simulink library "MET_lib"  (R2016b)
settings: Solver=VariableStepAuto  StartTime=0.0  StopTime=10.0  RelTol=1e-3
undefined symbols (not defined in the file or in its folder): sim_params
settings Model: Creator=taylorreynolds  LastModifiedBy=taylorreynolds

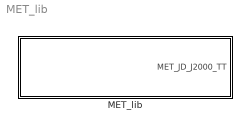
== system MET_lib ==
  MET_lib : Subsystem

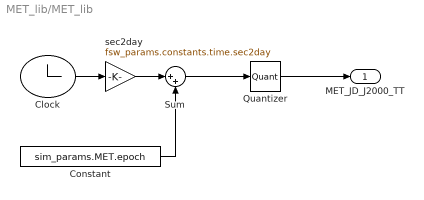
== system MET_lib/MET_lib ==
  Clock : Clock
  Constant : Constant  Value=sim_params.MET.epoch
  Quantizer : Quantizer  QuantizationInterval=sim_params.MET.res
  Sum : Sum  Inputs=|++
  sec2day : Gain  Gain=fsw_params.constants.time.sec2day
  MET_JD_J2000_TT : Outport
  wires:
  Clock/1 -> sec2day/1
  Constant/1 -> Sum/2
  Sum/1 -> Quantizer/1
  Quantizer/1 -> MET_JD_J2000_TT/1
  sec2day/1 -> Sum/1
